simulink model "Filtro_de_recepcao_5_4"  (R2013a)
settings: Solver=FixedStepDiscrete  StartTime=0.0  StopTime=800  RelTol=1e-3
values from neighbouring files (symbols this model uses):
  G = 0.1    [Variaveis.mat]
  T = 1    [Variaveis.mat]
undefined symbols (not defined in the file or in its folder): St
libraries: dspsigops x2
settings Model: Creator=Élio  LastModifiedBy=Élio

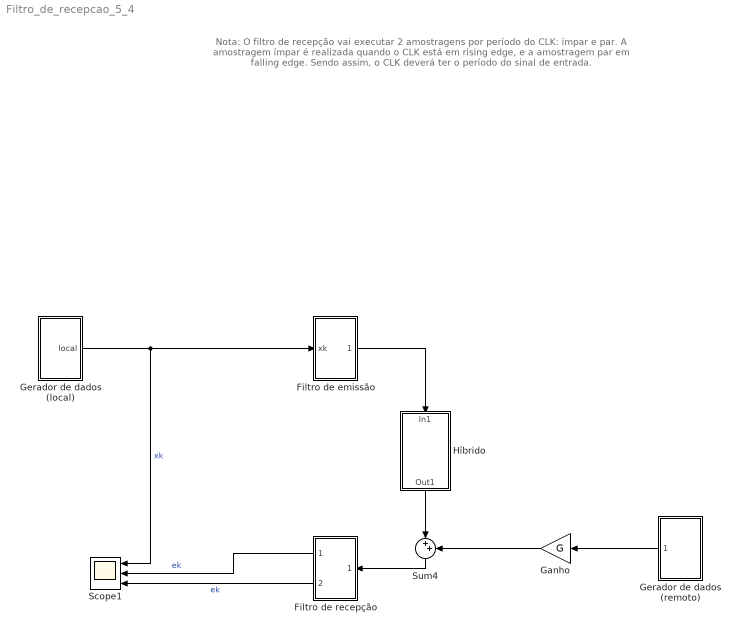
== system Filtro_de_recepcao_5_4 ==
  note: Nota: O filtro de recepção vai executar 2 amostragens
      | por período do CLK: ímpar e par. A amostragem ímpar
      | é realizada quando o CLK está em rising edge, e a
      | amostragem par em falling edge. Sendo assim, o CLK
      | deverá ter o período do sinal de entrada.
  "Filtro de emissão " : Subsystem
  Filtro de recepção : Subsystem
  Ganho : Gain  Gain=G
  Gerador de dados (local) : Subsystem
  Gerador de dados (remoto) : Subsystem
  Híbrido : Subsystem
  Scope1 : Scope  NumInputPorts=3
      settings: YMin=-5~-5~-5  YMax=5~5~5  SaveName=ScopeData3
  Sum4 : Sum  Inputs=|++
  wires:
  Gerador de dados (remoto)/1(remoto) -> Ganho/1
  Gerador de dados (local)/1(local) -> Scope1/1, "Filtro de emissão "/1(xk)  "xk"
  "Filtro de emissão "/1(Out1) -> Híbrido/1(In1)
  Híbrido/1(Out1) -> Sum4/1
  Ganho/1 -> Sum4/2
  Sum4/1 -> Filtro de recepção/1(In1)
  Filtro de recepção/1(ímpar) -> Scope1/2  "ek"
  Filtro de recepção/2(par) -> Scope1/3  "ek"

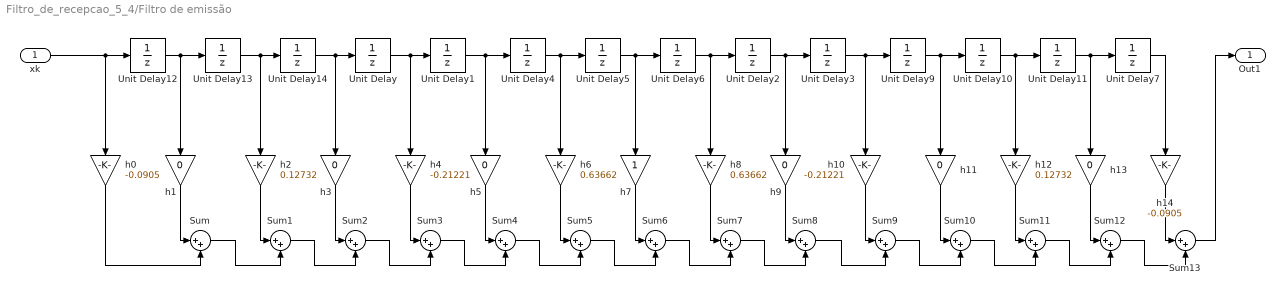
== system Filtro_de_recepcao_5_4/Filtro de emissão  ==
  xk : Inport
  Sum{,1..13} (14 alike) : Sum  Inputs=|++
  Unit Delay{,1..7,9..14} (14 alike) : UnitDelay  SampleTime=-1
  h0 : Gain  Gain=-0.0905
  h{1,3,5,9,11,13} (6 alike) : Gain  Gain=0
  h10 : Gain  Gain=-0.21221
  h12 : Gain  Gain=0.12732
  h14 : Gain  Gain=-0.0905
  h2 : Gain  Gain=0.12732
  h4 : Gain  Gain=-0.21221
  h6 : Gain  Gain=0.63662
  h7 : Gain
  h8 : Gain  Gain=0.63662
  Out1 : Outport
  wires:
  Unit Delay10/1 -> Unit Delay11/1, h12/1
  h3/1 -> Sum2/1
  Unit Delay1/1 -> Unit Delay4/1, h5/1
  h6/1 -> Sum5/1
  xk/1 -> Unit Delay12/1, h0/1
  Sum/1 -> Sum1/2
  h7/1 -> Sum6/1
  Unit Delay7/1 -> h14/1
  Unit Delay5/1 -> Unit Delay6/1, h7/1
  h5/1 -> Sum4/1
  h8/1 -> Sum7/1
  h9/1 -> Sum8/1
  h10/1 -> Sum9/1
  h1/1 -> Sum/1
  Unit Delay9/1 -> Unit Delay10/1, h11/1
  Unit Delay/1 -> Unit Delay1/1, h4/1
  Unit Delay12/1 -> Unit Delay13/1, h1/1
  Unit Delay4/1 -> Unit Delay5/1, h6/1
  Unit Delay2/1 -> Unit Delay3/1, h9/1
  Unit Delay3/1 -> Unit Delay9/1, h10/1
  Unit Delay11/1 -> Unit Delay7/1, h13/1
  h0/1 -> Sum/2
  Unit Delay6/1 -> Unit Delay2/1, h8/1
  Unit Delay13/1 -> Unit Delay14/1, h2/1
  h2/1 -> Sum1/1
  h4/1 -> Sum3/1
  Unit Delay14/1 -> Unit Delay/1, h3/1
  Sum13/1 -> Out1/1
  Sum12/1 -> Sum13/2
  Sum8/1 -> Sum9/2
  h11/1 -> Sum10/1
  h12/1 -> Sum11/1
  Sum4/1 -> Sum5/2
  Sum6/1 -> Sum7/2
  h14/1 -> Sum13/1
  Sum2/1 -> Sum3/2
  Sum11/1 -> Sum12/2
  Sum1/1 -> Sum2/2
  Sum9/1 -> Sum10/2
  h13/1 -> Sum12/1
  Sum3/1 -> Sum4/2
  Sum5/1 -> Sum6/2
  Sum10/1 -> Sum11/2
  Sum7/1 -> Sum8/2

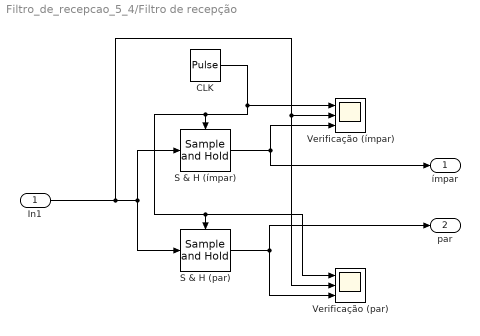
== system Filtro_de_recepcao_5_4/Filtro de recepção ==
  In1 : Inport
  CLK : DiscretePulseGenerator  PulseType=Time based  Period=2*T  PulseWidth=50  SampleTime=St
  "S & H (par) " : dspsigops/Sample and Hold  trig=Falling edge  initCond=0  latchinput=off
  "S & H (ímpar) " : dspsigops/Sample and Hold  trig=Rising edge  initCond=0  latchinput=off
  Verificação (par) : Scope  NumInputPorts=3
      settings: YMin=-5~-5~-5  YMax=5~5~5
  Verificação (ímpar) : Scope  NumInputPorts=3
      settings: YMin=-5~-5~-5  YMax=5~5~5
  ímpar : Outport
  par : Outport  Port=2
  wires:
  In1/1 -> Verificação (ímpar)/2, Verificação (par)/2, "S & H (ímpar) "/1, "S & H (par) "/1
  "S & H (ímpar) "/1 -> ímpar/1, Verificação (ímpar)/3
  "S & H (par) "/1 -> par/1, Verificação (par)/3
  CLK/1 -> Verificação (ímpar)/1, Verificação (par)/1, "S & H (par) "/Trigger, "S & H (ímpar) "/Trigger

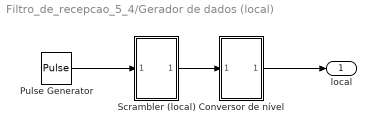
== system Filtro_de_recepcao_5_4/Gerador de dados (local) ==
  Conversor de nível : Subsystem
  Pulse Generator : DiscretePulseGenerator  PulseType=Time based  Period=2*T  PulseWidth=50  SampleTime=St
  Scrambler (local) : Subsystem
  local : Outport
  wires:
  Pulse Generator/1 -> Scrambler (local)/1(In1)
  Scrambler (local)/1(Out1) -> Conversor de nível/1(In2)
  Conversor de nível/1(Out2) -> local/1

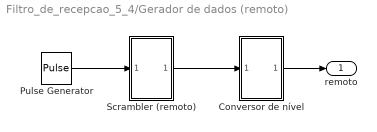
== system Filtro_de_recepcao_5_4/Gerador de dados (remoto) ==
  Conversor de nível : Subsystem
  Pulse Generator : DiscretePulseGenerator  PulseType=Time based  Period=2*T  PulseWidth=50  SampleTime=St
  Scrambler (remoto) : Subsystem
  remoto : Outport
  wires:
  Conversor de nível/1(Out2) -> remoto/1
  Scrambler (remoto)/1(Out1) -> Conversor de nível/1(In2)
  Pulse Generator/1 -> Scrambler (remoto)/1(In1)

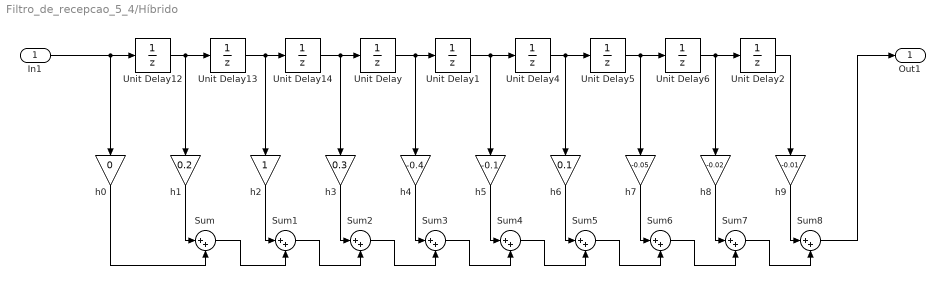
== system Filtro_de_recepcao_5_4/Híbrido ==
  In1 : Inport
  Sum{,1..8} (9 alike) : Sum  Inputs=|++
  Unit Delay{,1..2,4..6,12..14} (9 alike) : UnitDelay  SampleTime=-1
  h0 : Gain  Gain=0
  h1 : Gain  Gain=0.2
  h2 : Gain
  h3 : Gain  Gain=0.3
  h4 : Gain  Gain=-0.4
  h5 : Gain  Gain=-0.1
  h6 : Gain  Gain=0.1
  h7 : Gain  Gain=-0.05
  h8 : Gain  Gain=-0.02
  h9 : Gain  Gain=-0.01
  Out1 : Outport
  wires:
  In1/1 -> Unit Delay12/1, h0/1
  Unit Delay1/1 -> Unit Delay4/1, h5/1
  h2/1 -> Sum1/1
  h3/1 -> Sum2/1
  h6/1 -> Sum5/1
  h7/1 -> Sum6/1
  Sum/1 -> Sum1/2
  Unit Delay12/1 -> Unit Delay13/1, h1/1
  h4/1 -> Sum3/1
  h8/1 -> Sum7/1
  h9/1 -> Sum8/1
  h5/1 -> Sum4/1
  Sum1/1 -> Sum2/2
  Sum2/1 -> Sum3/2
  Unit Delay4/1 -> Unit Delay5/1, h6/1
  Unit Delay5/1 -> Unit Delay6/1, h7/1
  Unit Delay2/1 -> h9/1
  Unit Delay/1 -> Unit Delay1/1, h4/1
  Unit Delay14/1 -> Unit Delay/1, h3/1
  h1/1 -> Sum/1
  h0/1 -> Sum/2
  Unit Delay6/1 -> Unit Delay2/1, h8/1
  Unit Delay13/1 -> Unit Delay14/1, h2/1
  Sum3/1 -> Sum4/2
  Sum5/1 -> Sum6/2
  Sum8/1 -> Out1/1
  Sum4/1 -> Sum5/2
  Sum7/1 -> Sum8/2
  Sum6/1 -> Sum7/2

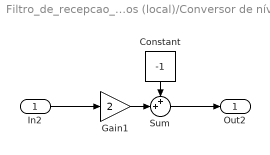
== system Filtro_de_recepcao_5_4/Gerador de dados (local)/Conversor de nível ==
  In2 : Inport
  Constant : Constant  Value=-1
  Gain1 : Gain  Gain=2
  Sum : Sum  Inputs=++|
  Out2 : Outport
  wires:
  In2/1 -> Gain1/1
  Sum/1 -> Out2/1
  Gain1/1 -> Sum/2
  Constant/1 -> Sum/1

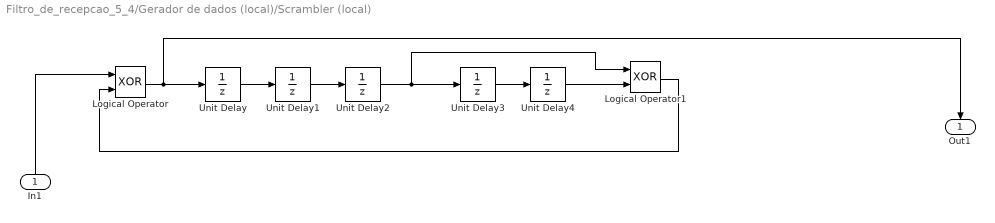
== system Filtro_de_recepcao_5_4/Gerador de dados (local)/Scrambler (local) ==
  In1 : Inport
  Logical Operator : Logic  Operator=XOR  AllPortsSameDT=off  OutDataTypeStr=fixdt(1,16)
  Logical Operator1 : Logic  Operator=XOR  AllPortsSameDT=off  OutDataTypeStr=boolean
  Unit Delay{,1..4} (5 alike) : UnitDelay  SampleTime=-1
  Out1 : Outport
  wires:
  In1/1 -> Logical Operator/1
  Logical Operator/1 -> Out1/1, Unit Delay/1
  Unit Delay/1 -> Unit Delay1/1
  Logical Operator1/1 -> Logical Operator/2
  Unit Delay3/1 -> Unit Delay4/1
  Unit Delay4/1 -> Logical Operator1/2
  Unit Delay1/1 -> Unit Delay2/1
  Unit Delay2/1 -> Logical Operator1/1, Unit Delay3/1

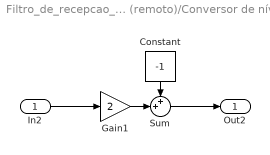
== system Filtro_de_recepcao_5_4/Gerador de dados (remoto)/Conversor de nível ==
  In2 : Inport
  Constant : Constant  Value=-1
  Gain1 : Gain  Gain=2
  Sum : Sum  Inputs=++|
  Out2 : Outport
  wires:
  In2/1 -> Gain1/1
  Sum/1 -> Out2/1
  Gain1/1 -> Sum/2
  Constant/1 -> Sum/1

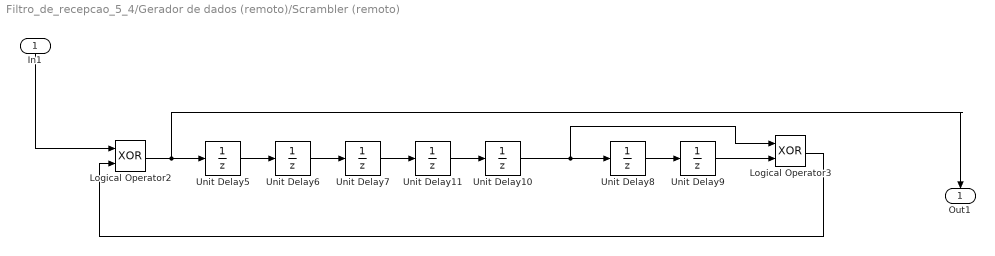
== system Filtro_de_recepcao_5_4/Gerador de dados (remoto)/Scrambler (remoto) ==
  In1 : Inport
  Logical Operator2 : Logic  Operator=XOR  AllPortsSameDT=off  OutDataTypeStr=fixdt(1,16)
  Logical Operator3 : Logic  Operator=XOR  AllPortsSameDT=off  OutDataTypeStr=boolean
  Unit Delay{5..11} (7 alike) : UnitDelay  SampleTime=-1
  Out1 : Outport
  wires:
  In1/1 -> Logical Operator2/1
  Unit Delay6/1 -> Unit Delay7/1
  Unit Delay9/1 -> Logical Operator3/2
  Unit Delay11/1 -> Unit Delay10/1
  Unit Delay10/1 -> Logical Operator3/1, Unit Delay8/1
  Logical Operator3/1 -> Logical Operator2/2
  Unit Delay7/1 -> Unit Delay11/1
  Unit Delay8/1 -> Unit Delay9/1
  Logical Operator2/1 -> Out1/1, Unit Delay5/1
  Unit Delay5/1 -> Unit Delay6/1
